simulink model "controlador_interno_sist_completo_NL"  (R2019a)
settings: Solver=VariableStepAuto  StartTime=0.0  StopTime=10.0  RelTol=1e-3
undefined symbols (not defined in the file): alpha_cu, b_eq, C_ts, J_eq, L_d, L_ls, L_q, lambda_m, P_p, r, R_0, R_d, R_q, R_s_40, R_ts_amb
libraries: eeTransforms x4
settings Model: Creator=miact  LastModifiedBy=miact

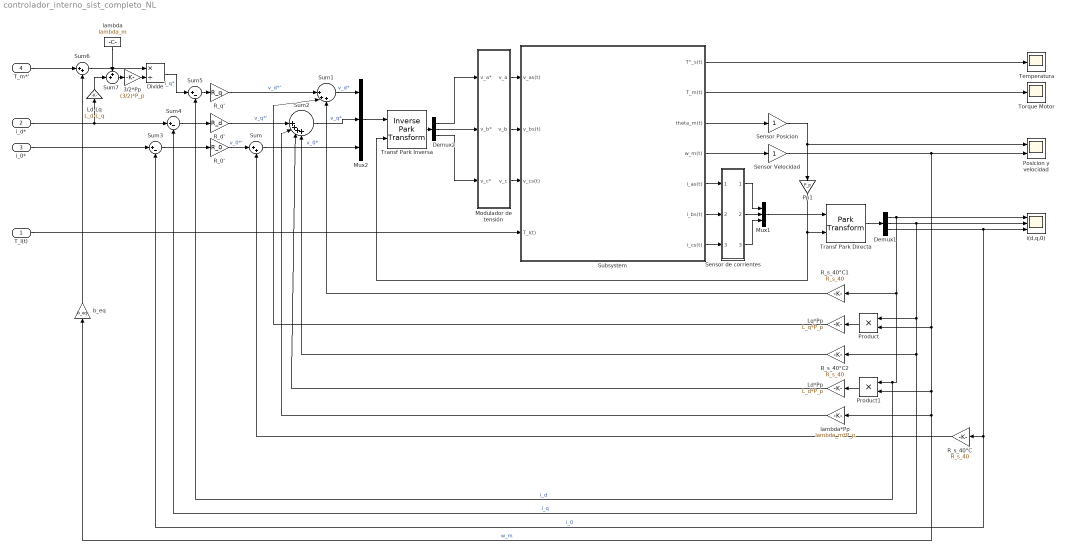
== system controlador_interno_sist_completo_NL ==
  T_l(t) : Inport
  i_d* : Inport  Port=2
  i_0* : Inport  Port=3
  T_m*' : Inport  Port=4
  3/2*Pp : Gain  Gain=(3/2)*P_p
  Demux1 : Demux  Outputs=3
  Demux2 : Demux  Outputs=3
  Divide : Product  Inputs=*/
  Ld*Pp : Gain  Gain=L_d*P_p
  "Ld-Lq " : Gain  Gain=L_d-L_q
  Lq*Pp : Gain  Gain=L_q*P_p
  Modulador de tensión : Subsystem
  Mux1 : Mux  Inputs=3
  Mux2 : Mux  Inputs=3
  Posicion y velocidad : Scope  NumInputPorts=2
  Pp1 : Gain  Gain=P_p
  Product : Product
  Product1 : Product
  "R_0' " : Gain  Gain=R_0
  R_d' : Gain  Gain=R_d
  R_q' : Gain  Gain=R_q
  R_s_40°C : Gain  Gain=R_s_40
  R_s_40°C1 : Gain  Gain=R_s_40
  R_s_40°C2 : Gain  Gain=R_s_40
  Sensor Posicion : Gain
  Sensor Velocidad : Gain
  Sensor de corrientes : Subsystem
  Subsystem : Subsystem
  Sum : Sum  Inputs=|++
  Sum1 : Sum  Inputs=||+++
  Sum2 : Sum  Inputs=|||++++
  Sum3 : Sum  Inputs=|+-
  Sum4 : Sum  Inputs=|+-
  Sum5 : Sum  Inputs=|+-
  Sum6 : Sum  Inputs=|++
  Sum7 : Sum  Inputs=++|
  Temperatura : Scope
  Torque Motor : Scope
  Transf Park Inversa : eeTransforms/Inverse Park Transform  AxisAlignment=Q-axis  PowerInvariant=off
      settings: SourceProductName=Simscape Electrical
  Transf Park Directa : eeTransforms/Park Transform  AxisAlignment=Q-axis  PowerInvariant=off
      settings: SourceProductName=Simscape Electrical
  b_eq : Gain  Gain=b_eq
  "i(d,q,0) " : Scope  NumInputPorts=3
  lambda : Constant  Value=lambda_m
  lambda*Pp : Gain  Gain=lambda_m*P_p
  wires:
  Subsystem/1(T°_s(t)) -> Temperatura/1
  Subsystem/2("T_m(t) ") -> Torque Motor/1
  Subsystem/5(i_as(t)) -> Sensor de corrientes/1("I_a ")
  Subsystem/6(i_bs(t)) -> Sensor de corrientes/2(I_b)
  Subsystem/7(i_cs(t)) -> Sensor de corrientes/3(I_c)
  Subsystem/3(theta_m(t)) -> Sensor Posicion/1
  Sensor Posicion/1 -> Posicion y velocidad/1, Pp1/1
  Subsystem/4(w_m(t)) -> Sensor Velocidad/1
  Sensor Velocidad/1 -> b_eq/1, lambda*Pp/1, Product1/2, Product/2, Posicion y velocidad/2  "w_m"
  Mux1/1 -> Transf Park Directa/1
  Sensor de corrientes/1(i_a) -> Mux1/1
  Sensor de corrientes/2(i_b) -> Mux1/2
  Sensor de corrientes/3(i_c) -> Mux1/3
  Transf Park Directa/1 -> Demux1/1
  Pp1/1 -> Transf Park Directa/2, Transf Park Inversa/2
  Modulador de tensión/1(v_a) -> Subsystem/1(v_as(t))
  Modulador de tensión/2(v_b) -> Subsystem/2(v_bs(t))
  Modulador de tensión/3(v_c) -> Subsystem/3(v_cs(t))
  Transf Park Inversa/1 -> Demux2/1
  Demux2/1 -> Modulador de tensión/1(v_a*)
  Demux2/2 -> Modulador de tensión/2(v_b*)
  Demux2/3 -> Modulador de tensión/3(v_c*)
  Mux2/1 -> Transf Park Inversa/1
  Demux1/3 -> "i(d,q,0) "/3, R_s_40°C/1, Sum3/2  "i_0"
  Sum/1 -> Mux2/3  "v_0*"
  R_s_40°C/1 -> Sum/2
  Demux1/1 -> "i(d,q,0) "/1, R_s_40°C1/1, Product1/1, Sum5/2  "i_d"
  Sum1/1 -> Mux2/1  "v_d*"
  R_s_40°C1/1 -> Sum1/3
  Demux1/2 -> R_s_40°C2/1, Sum4/2, Product/1, "i(d,q,0) "/2  "i_q"
  Product/1 -> Lq*Pp/1
  Lq*Pp/1 -> Sum1/2
  Sum2/1 -> Mux2/2  "v_q*"
  R_s_40°C2/1 -> Sum2/4
  Product1/1 -> Ld*Pp/1
  Ld*Pp/1 -> Sum2/3
  lambda*Pp/1 -> Sum2/2
  R_q'/1 -> Sum1/1  "v_d*'"
  R_d'/1 -> Sum2/1  "v_q*'"
  "R_0' "/1 -> Sum/1  "v_0*'"
  Sum3/1 -> "R_0' "/1
  Sum4/1 -> R_d'/1
  Sum5/1 -> R_q'/1
  Divide/1 -> Sum5/1  "i_q*"
  T_l(t)/1 -> Subsystem/4(T_l(t))
  i_0*/1 -> Sum3/1
  Sum6/1 -> Divide/1
  3/2*Pp/1 -> Divide/2
  Sum7/1 -> 3/2*Pp/1
  lambda/1 -> Sum7/1
  "Ld-Lq "/1 -> Sum7/2
  i_d*/1 -> "Ld-Lq "/1, Sum4/1
  b_eq/1 -> Sum6/2
  T_m*'/1 -> Sum6/1

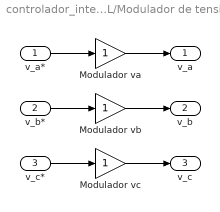
== system controlador_interno_sist_completo_NL/Modulador de tensión ==
  v_a* : Inport
  v_b* : Inport  Port=2
  v_c* : Inport  Port=3
  Modulador va : Gain
  Modulador vb : Gain
  Modulador vc : Gain
  v_a : Outport
  v_b : Outport  Port=2
  v_c : Outport  Port=3
  wires:
  v_c*/1 -> Modulador vc/1
  Modulador va/1 -> v_a/1
  v_b*/1 -> Modulador vb/1
  Modulador vb/1 -> v_b/1
  Modulador vc/1 -> v_c/1
  v_a*/1 -> Modulador va/1

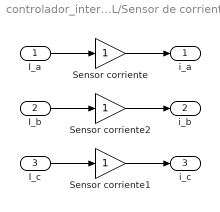
== system controlador_interno_sist_completo_NL/Sensor de corrientes ==
  "I_a " : Inport
  I_b : Inport  Port=2
  I_c : Inport  Port=3
  Sensor corriente : Gain
  Sensor corriente1 : Gain
  Sensor corriente2 : Gain
  i_a : Outport
  i_b : Outport  Port=2
  i_c : Outport  Port=3
  wires:
  I_c/1 -> Sensor corriente1/1
  Sensor corriente/1 -> i_a/1
  I_b/1 -> Sensor corriente2/1
  Sensor corriente2/1 -> i_b/1
  Sensor corriente1/1 -> i_c/1
  "I_a "/1 -> Sensor corriente/1

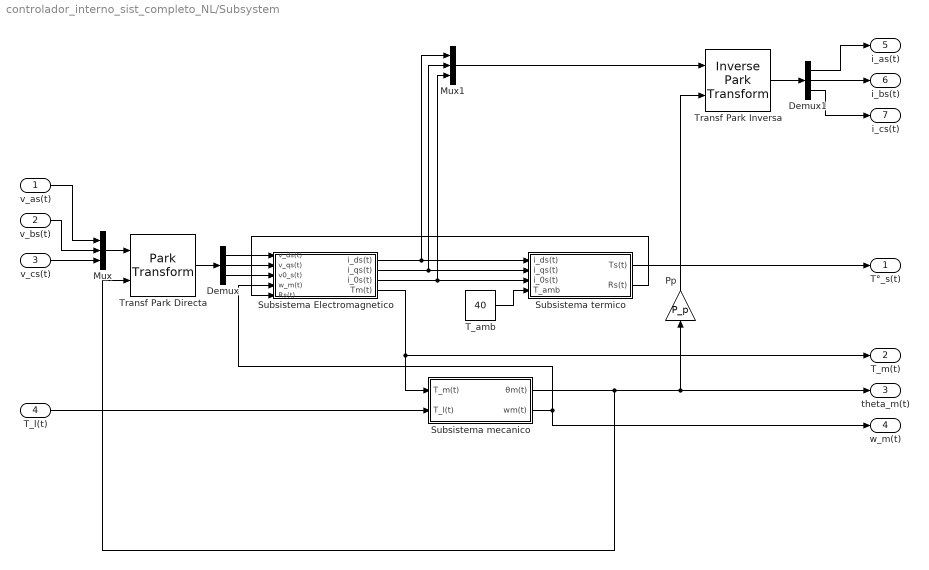
== system controlador_interno_sist_completo_NL/Subsystem ==
  v_as(t) : Inport
  v_bs(t) : Inport  Port=2
  v_cs(t) : Inport  Port=3
  T_l(t) : Inport  Port=4
  Demux : Demux  Outputs=3
  Demux1 : Demux  Outputs=3
  Mux : Mux  Inputs=3
  Mux1 : Mux  Inputs=3
  Pp : Gain  Gain=P_p
  Subsistema Electromagnetico : Subsystem
  "Subsistema mecanico " : Subsystem
  "Subsistema termico " : Subsystem
  T_amb : Constant  Value=40
  Transf Park Inversa : eeTransforms/Inverse Park Transform  AxisAlignment=Q-axis  PowerInvariant=off
      settings: SourceProductName=Simscape Electrical
  Transf Park Directa : eeTransforms/Park Transform  AxisAlignment=Q-axis  PowerInvariant=off
      settings: SourceProductName=Simscape Electrical
  T°_s(t) : Outport
  "T_m(t) " : Outport  Port=2
  theta_m(t) : Outport  Port=3
  w_m(t) : Outport  Port=4
  i_as(t) : Outport  Port=5
  i_bs(t) : Outport  Port=6
  i_cs(t) : Outport  Port=7
  wires:
  T_amb/1 -> "Subsistema termico "/4(T_amb)
  "Subsistema termico "/2(Rs(t)) -> Subsistema Electromagnetico/5("Rs(t) ")
  "Subsistema termico "/1(Ts(t)) -> T°_s(t)/1
  Subsistema Electromagnetico/2("i_qs(t) ") -> Mux1/2, "Subsistema termico "/2("i_qs(t) ")
  "Subsistema mecanico "/2(wm(t)) -> w_m(t)/1, Subsistema Electromagnetico/4(w_m(t))
  Subsistema Electromagnetico/1(i_ds(t)) -> Mux1/1, "Subsistema termico "/1("i_ds(t) ")
  Subsistema Electromagnetico/3("i_0s(t) ") -> Mux1/3, "Subsistema termico "/3(i_0s(t))
  "Subsistema mecanico "/1(θm(t)) -> Transf Park Directa/2, Pp/1, theta_m(t)/1
  Pp/1 -> Transf Park Inversa/2
  T_l(t)/1 -> "Subsistema mecanico "/2("T_l(t) ")
  Mux/1 -> Transf Park Directa/1
  v_as(t)/1 -> Mux/1
  v_bs(t)/1 -> Mux/2
  v_cs(t)/1 -> Mux/3
  Transf Park Directa/1 -> Demux/1
  Demux/3 -> Subsistema Electromagnetico/3(v0_s(t))
  Mux1/1 -> Transf Park Inversa/1
  Subsistema Electromagnetico/4(Tm(t)) -> "Subsistema mecanico "/1("T_m(t) "), "T_m(t) "/1
  Transf Park Inversa/1 -> Demux1/1
  Demux1/1 -> i_as(t)/1
  Demux1/2 -> i_bs(t)/1
  Demux1/3 -> i_cs(t)/1
  Demux/1 -> Subsistema Electromagnetico/1(v_ds(t))
  Demux/2 -> Subsistema Electromagnetico/2(v_qs(t))

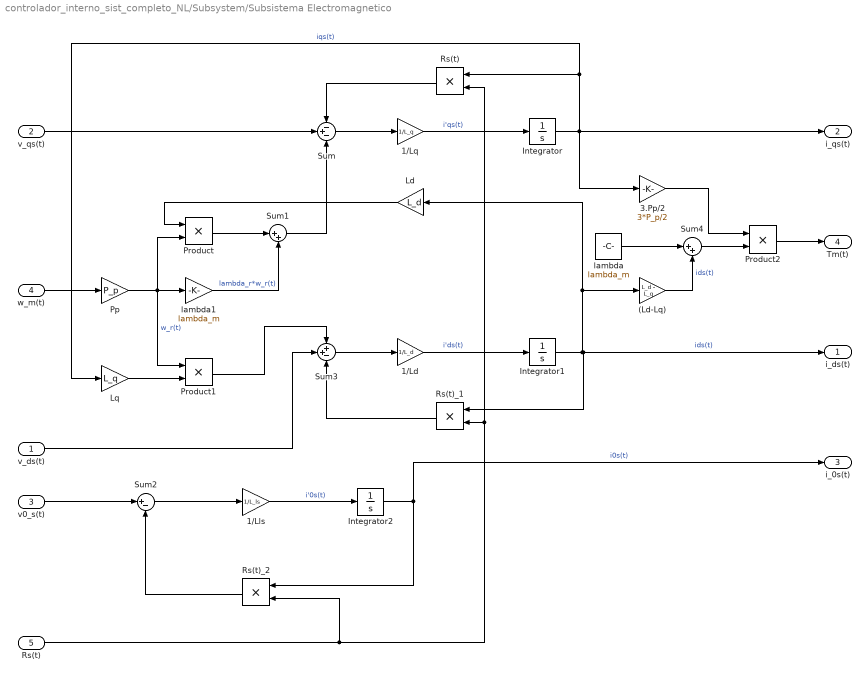
== system controlador_interno_sist_completo_NL/Subsystem/Subsistema Electromagnetico ==
  v_ds(t) : Inport
  v_qs(t) : Inport  Port=2
  v0_s(t) : Inport  Port=3
  w_m(t) : Inport  Port=4
  "Rs(t) " : Inport  Port=5
  (Ld-Lq) : Gain  Gain=L_d - L_q
  1/Ld : Gain  Gain=1/L_d
  1/Lls : Gain  Gain=1/L_ls
  1/Lq : Gain  Gain=1/L_q
  3.Pp/2 : Gain  Gain=3*P_p/2
  Integrator : Integrator
  Integrator1 : Integrator
  Integrator2 : Integrator
  Ld : Gain  Gain=L_d
  Lq : Gain  Gain=L_q
  Pp : Gain  Gain=P_p
  Product : Product
  Product1 : Product
  Product2 : Product
  Rs(t) : Product
  Rs(t)_1 : Product
  Rs(t)_2 : Product
  Sum : Sum  Inputs=-+-
  Sum1 : Sum  Inputs=|++
  Sum2 : Sum  Inputs=|+-
  Sum3 : Sum  Inputs=++-
  Sum4 : Sum  Inputs=|++
  lambda : Constant  Value=lambda_m
  lambda1 : Gain  Gain=lambda_m
  i_ds(t) : Outport
  "i_qs(t) " : Outport  Port=2
  "i_0s(t) " : Outport  Port=3
  Tm(t) : Outport  Port=4
  wires:
  w_m(t)/1 -> Pp/1
  Pp/1 -> Product1/1, Product/2, lambda1/1  "w_r(t)"
  Sum/1 -> 1/Lq/1
  1/Lq/1 -> Integrator/1  "i'qs(t)"
  Sum1/1 -> Sum/3
  v_qs(t)/1 -> Sum/2
  Integrator/1 -> Lq/1, Rs(t)/1, 3.Pp/2/1, "i_qs(t) "/1  "iqs(t)"
  lambda1/1 -> Sum1/2  "lambda_r*w_r(t)"
  Product/1 -> Sum1/1
  v_ds(t)/1 -> Sum3/2
  Sum3/1 -> 1/Ld/1
  Product1/1 -> Sum3/1
  1/Ld/1 -> Integrator1/1  "i'ds(t)"
  Integrator1/1 -> Ld/1, (Ld-Lq)/1, Rs(t)_1/1, i_ds(t)/1  "ids(t)"
  Lq/1 -> Product1/2
  Ld/1 -> Product/1
  v0_s(t)/1 -> Sum2/1
  Rs(t)_2/1 -> Sum2/2
  Sum2/1 -> 1/Lls/1
  1/Lls/1 -> Integrator2/1  "i'0s(t)"
  Integrator2/1 -> Rs(t)_2/1, "i_0s(t) "/1  "i0s(t)"
  (Ld-Lq)/1 -> Sum4/2  "ids(t)"
  lambda/1 -> Sum4/1
  Sum4/1 -> Product2/2
  Product2/1 -> Tm(t)/1
  3.Pp/2/1 -> Product2/1
  "Rs(t) "/1 -> Rs(t)_2/2, Rs(t)/2, Rs(t)_1/2
  Rs(t)_1/1 -> Sum3/3
  Rs(t)/1 -> Sum/1

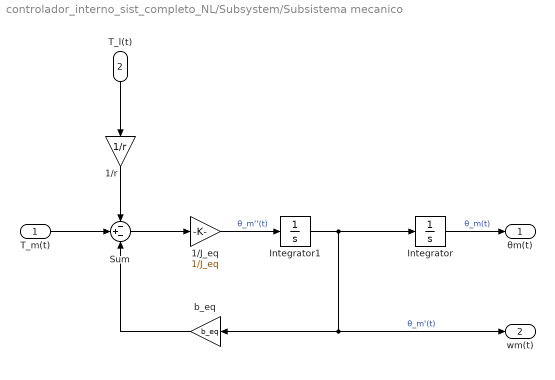
== system controlador_interno_sist_completo_NL/Subsystem/Subsistema mecanico  ==
  "T_m(t) " : Inport
  "T_l(t) " : Inport  Port=2
  "1/J_eq " : Gain  Gain=1/J_eq
  1/r : Gain  Gain=1/r
  Integrator : Integrator
  Integrator1 : Integrator
  Sum : Sum  Inputs=-+-
  b_eq : Gain  Gain=b_eq
  θm(t) : Outport
  wm(t) : Outport  Port=2
  wires:
  Integrator1/1 -> b_eq/1, wm(t)/1, Integrator/1  "θ_m'(t)"
  Sum/1 -> "1/J_eq "/1
  b_eq/1 -> Sum/3
  "1/J_eq "/1 -> Integrator1/1  "θ_m''(t)"
  Integrator/1 -> θm(t)/1  "θ_m(t)"
  "T_m(t) "/1 -> Sum/2
  "T_l(t) "/1 -> 1/r/1
  1/r/1 -> Sum/1

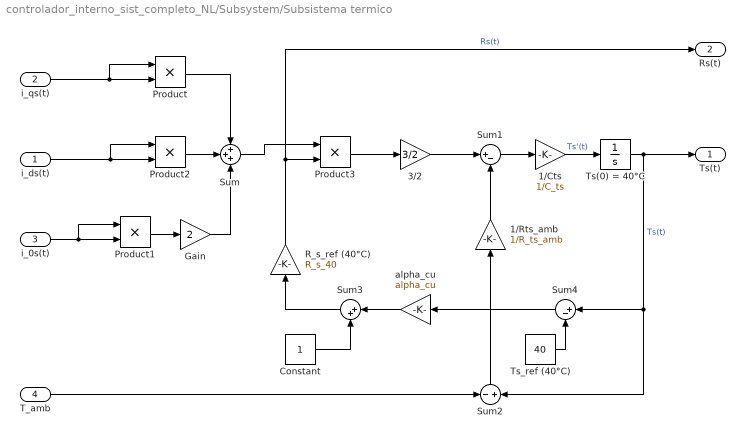
== system controlador_interno_sist_completo_NL/Subsystem/Subsistema termico  ==
  "i_ds(t) " : Inport
  "i_qs(t) " : Inport  Port=2
  i_0s(t) : Inport  Port=3
  T_amb : Inport  Port=4
  1/Cts : Gain  Gain=1/C_ts
  1/Rts_amb : Gain  Gain=1/R_ts_amb
  3/2 : Gain  Gain=3/2
  Constant : Constant
  Gain : Gain  Gain=2
  Product{,1..3} (4 alike) : Product
  R_s_ref (40°C) : Gain  Gain=R_s_40
  Sum : Sum  Inputs=+++
  Sum1 : Sum  Inputs=|+-
  Sum2 : Sum  Inputs=-|+
  Sum3 : Sum  Inputs=|++
  Sum4 : Sum  Inputs=|+-
  Ts(0) = 40°C : Integrator  InitialCondition=40
  Ts_ref (40°C) : Constant  Value=40
  alpha_cu : Gain  Gain=alpha_cu
  Ts(t) : Outport
  Rs(t) : Outport  Port=2
  wires:
  i_0s(t)/1 -> Product1/1, Product1/2
  "i_ds(t) "/1 -> Product2/1, Product2/2
  "i_qs(t) "/1 -> Product/1, Product/2
  Product/1 -> Sum/1
  Product2/1 -> Sum/2
  Ts(0) = 40°C/1 -> Sum4/1, Sum2/2, Ts(t)/1  "Ts(t)"
  T_amb/1 -> Sum2/1
  Sum2/1 -> 1/Rts_amb/1
  1/Rts_amb/1 -> Sum1/2
  Sum1/1 -> 1/Cts/1
  1/Cts/1 -> Ts(0) = 40°C/1  "Ts'(t)"
  Constant/1 -> Sum3/2
  alpha_cu/1 -> Sum3/1
  Sum3/1 -> R_s_ref (40°C)/1
  R_s_ref (40°C)/1 -> Rs(t)/1, Product3/2  "Rs(t)"
  Sum/1 -> Product3/1
  Product3/1 -> 3/2/1
  3/2/1 -> Sum1/1
  Ts_ref (40°C)/1 -> Sum4/2
  Sum4/1 -> alpha_cu/1
  Gain/1 -> Sum/3
  Product1/1 -> Gain/1
